simulink model "Vehicle_Performance_Model_range"  (R2020a)
settings: Solver=FixedStepAuto  StartTime=0  StopTime=50000000  FixedStep=time_step  RelTol=1e-3
values from neighbouring files (symbols this model uses):
  battery_capacity = 40000    [aa_main_code.m]
  BrkGain = 1e4    (= 10000)    [HW5_Initialization.m]    (also in aa_main_code.m; aa_main_code_optimization.m)
  Cd = 0.27    [aa_main_code.m]    (also in aa_main_code_optimization.m)
  CG_a = (mass_x_dis/mass_CG) - L104    [aa_main_code.m]    (also in aa_main_code_optimization.m)
  CG_b = L101 - CG_a    [aa_main_code.m]    (also in aa_main_code_optimization.m)
  CG_h = mass_Y_dis/mass_CG    [aa_main_code.m]    (also in aa_main_code_optimization.m)
  Cr = 0.009    [aa_main_code.m]    (also in aa_main_code_optimization.m)
  drive_ratio = 2    [aa_main_code.m]
  eff_dl = 0.9    [HW5_Initialization.m]    (also in aa_main_code.m; aa_main_code_optimization.m)
  EM_Efficiency = [0.85 0.7 0.7 0.7 0.69 0.65 0.6 0.55 0.55 0.55 0.55 0.55 ... (854 elements, 14x61)]    [MotorA_Data.mat]    (also in MotorB_Data.mat = [0.1063790939 0.270163202936 0.172582128791 0.0795422183598 ; MotorC_Data.mat = [0.156591344269 0.267837551 0.221914755199 0.160062614994 0.)
  EM_Omega_Max = [0 38.3972435439 76.7944870878 115.191730632 153.588974176 191.986217719 203.505390783 230.383461263 268.780704807 307.177948351 326.376570123 345.575191895 ... (24 elements, 1x24)]    [MotorA_Data.mat]    (also in MotorB_Data.mat = [0 334.056952995 360.213537682 388.612115341 414.768700028 4; MotorC_Data.mat = [0 130.235063563 190.672775215 254.736749566 349.019579743 3)
  EM_Torque_Max = [765 765 765 765 765 765 765 765 765 765 765 722.5 ... (24 elements, 1x24)]    [MotorA_Data.mat]    (also in MotorB_Data.mat = [300 300 279.372738239 258.745476478 241.737032569 222.55729; MotorC_Data.mat = [420 420 420 420 420 400.59405651 375.297526478 350.00099644)
  front_on = 1    [aa_main_code.m]    (also in aa_main_code_optimization.m)
  g = 9.81    [HW5_Initialization.m]    (also in aa_main_code.m; aa_main_code_optimization.m)
  Ki = 1    [HW5_Initialization.m]    (also in aa_main_code.m = 0.03; aa_main_code_optimization.m = 0.03)
  Kp = 3    [HW5_Initialization.m]    (also in aa_main_code.m = 0.5; aa_main_code_optimization.m = 0.5)
  L101 = 2700/1000    (= 2.7)    [aa_main_code.m]    (also in aa_main_code_optimization.m)
  m = 2000    [HW5_Initialization.m]
  mass = (4*passenger_mass)+cargo_mass+info_mass+sunroof_mass+unsprung_mass+total_gearbox_mass+total_differential_mass+axle_mass+body_mass+frame_rail_mass+battery_mass+total_motorinverter_mass    (= 1622.8836992)    [aa_main_code.m]    (also in aa_main_code_optimization.m = (4*passenger_mass)+cargo_mass+info_mass+sunroof_mass+unsprun)
  mu = 0.9    [HW5_Initialization.m]    (also in aa_main_code.m; aa_main_code_optimization.m)
  num_motor = 4    [aa_main_code.m]    (also in aa_main_code_optimization.m)
  omega_BP = max(size(EM_Omega_Map))    [aa_main_code.m]    (also in aa_main_code_optimization.m)
  omega_max = max(EM_Omega_Max)    [aa_main_code.m]    (also in aa_main_code_optimization.m)
  r = 0.335    [HW5_Initialization.m]    (also in aa_main_code.m = 0.32985; aa_main_code_optimization.m = 0.32985)
  rear_on = 1    [aa_main_code.m]    (also in aa_main_code_optimization.m)
  rho = 1.3    [HW5_Initialization.m]    (also in aa_main_code.m = 1.26; aa_main_code_optimization.m = 1.26)
  slope = 0.12    [aa_main_code.m]    (also in aa_main_code_optimization.m)
  torque_BP = max(size(EM_Torque_Map))    [aa_main_code.m]    (also in aa_main_code_optimization.m)
  torque_multi_factor = 2    [aa_main_code.m]    (also in aa_main_code_optimization.m)
  useful_battery_capacity = 0.95    [aa_main_code.m]    (also in aa_main_code_optimization.m)
  vehicle_frontal_area = H101*W103    (= 2.5844)    [aa_main_code.m]    (also in aa_main_code_optimization.m)
libraries: simulink x5, autolibshared x1
settings Model: Creator=palak  LastModifiedBy=atefe
settings SolverCC: AlgebraicLoopSolver=LineSearch

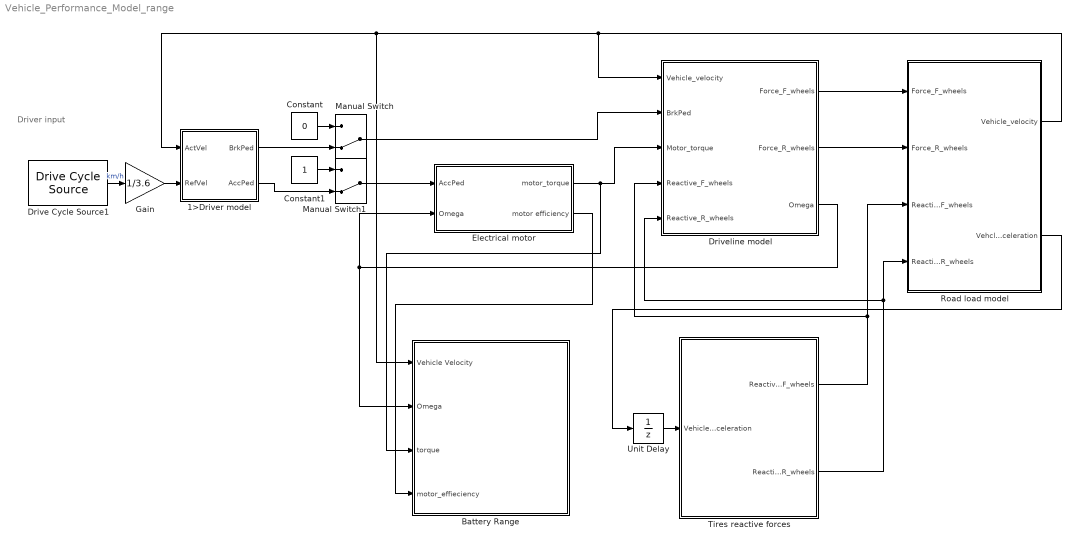
== system Vehicle_Performance_Model_range ==
  note: Driver input
  1>Driver model : Subsystem
  Battery Range : Subsystem
  Constant : Constant  Value=0
  Constant1 : Constant
  Drive Cycle Source1 : autolibshared/Drive Cycle Source  cycleVar=Workspace variable  wsVar=cycle  fileVar=cycleFTP75.mat  tfinal="600  seconds, Cyclic"  cycleRepeat=on  outAccPort=off  outGearPort=off  gearList=No gear data  t_wot1=5  xdot_woto=0  xdot_wot1=30  t_wot2=20  xdot_wot2=0  t_wotend=30  srcUnit=m/s  outUnit=m/s  srcAccUnit=m/s/s  outAccUnit=m/s^2  dt=0  aMode=1  faultOption=off  velBnd=2  velBndUnit=mph  inUnit=m/s  timeBnd=1  failOption=off  stopSim=off  maxFaultCnt=10  maxFaultTime=2  maxTotFaultTime=15  traceOption=off  dtTrace=1  traceWindow=10  lastDCname=Custom Data Set  lastOutUnit=mph  lastDT=0  lastTB=1  lastSB=2  forceCalcBound=off
      settings: SourceProductBaseCode=PW,MT,VE,VP
  Driveline model : Subsystem
  Electrical motor : Subsystem
  Gain : Gain  Gain=1/3.6
  Manual Switch : ManualSwitch  CurrentSetting=0
  Manual Switch1 : ManualSwitch  CurrentSetting=0
  Road load model : Subsystem
  Tires reactive forces : Subsystem  TreatAsAtomicUnit=on
  Unit Delay : UnitDelay  SampleTime=-1  HasFrameUpgradeWarning=on
  wires:
  Gain/1 -> 1>Driver model/2(RefVel)
  Driveline model/3(Omega) -> Electrical motor/2(Omega), Battery Range/2(Omega)
  Road load model/1(Vehicle_velocity) -> Driveline model/1(Vehicle_velocity), Battery Range/1(Vehicle Velocity), 1>Driver model/1(ActVel)
  Driveline model/1(Force_F_wheels) -> Road load model/1(Force_F_wheels)
  Manual Switch/1 -> Driveline model/2(BrkPed)
  Electrical motor/1(motor_torque) -> Battery Range/3(torque), Driveline model/3(Motor_torque)
  Road load model/2(Vehcle_acceleration) -> Unit Delay/1
  Tires reactive forces/1(Reactive_F_wheels) -> Road load model/3(Reactive_F_wheels), Driveline model/4(Reactive_F_wheels)
  Tires reactive forces/2(Reactive_R_wheels) -> Road load model/4(Reactive_R_wheels), Driveline model/5(Reactive_R_wheels)
  Driveline model/2(Force_R_wheels) -> Road load model/2(Force_R_wheels)
  Electrical motor/2(motor efficiency) -> Battery Range/4(motor_effieciency)
  Drive Cycle Source1/1 -> Gain/1  "km/h"
  Manual Switch1/1 -> Electrical motor/1(AccPed)
  1>Driver model/1(BrkPed) -> Manual Switch/2
  Constant/1 -> Manual Switch/1
  Constant1/1 -> Manual Switch1/1
  1>Driver model/2(AccPed) -> Manual Switch1/2
  Unit Delay/1 -> Tires reactive forces/1(Vehicle_acceleration)

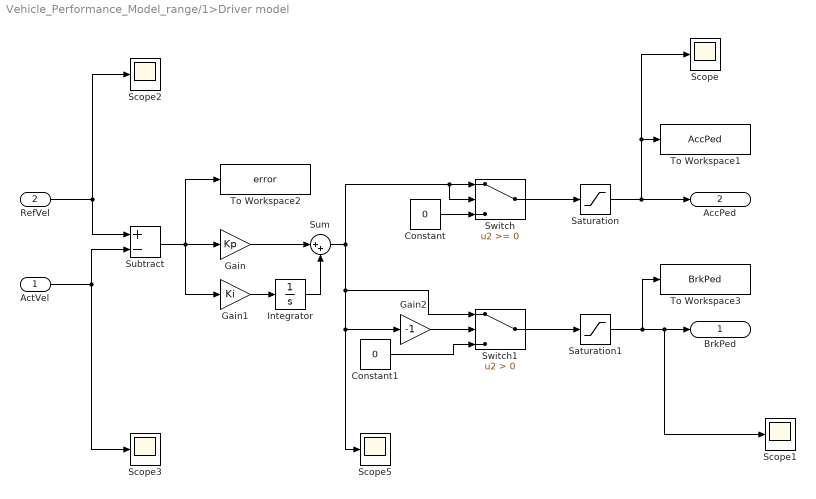
== system Vehicle_Performance_Model_range/1>Driver model ==
  ActVel : Inport  Unit=m/s
  RefVel : Inport  Port=2  Unit=m/s
  Constant : Constant  Value=0
  Constant1 : Constant  Value=0
  Gain : Gain  Gain=Kp
  Gain1 : Gain  Gain=Ki
  Gain2 : Gain  Gain=-1
  Integrator : Integrator
  Saturation : Saturate  UpperLimit=1  LowerLimit=0
  Saturation1 : Saturate  UpperLimit=0  LowerLimit=-1
  Scope{,1..3,5} (5 alike) : Scope
  Subtract : Sum  Inputs=+-
  Sum : Sum  Inputs=|++
  Switch : Switch
  Switch1 : Switch  Criteria=u2 > Threshold
  To Workspace1 : ToWorkspace  VariableName=AccPed  SaveFormat=Timeseries  SampleTime=-1
  To Workspace2 : ToWorkspace  VariableName=error  SaveFormat=Timeseries  SampleTime=-1
  To Workspace3 : ToWorkspace  VariableName=BrkPed  SaveFormat=Timeseries  SampleTime=-1
  BrkPed : Outport
  AccPed : Outport  Port=2
  wires:
  ActVel/1 -> Scope3/1, Subtract/2
  RefVel/1 -> Scope2/1, Subtract/1
  Saturation/1 -> Scope/1, To Workspace1/1, AccPed/1
  Sum/1 -> Scope5/1, Gain2/1, Switch1/1, Switch/2, Switch/1
  Subtract/1 -> Gain1/1, Gain/1, To Workspace2/1
  Gain/1 -> Sum/1
  Integrator/1 -> Sum/2
  Gain1/1 -> Integrator/1
  Constant/1 -> Switch/3
  Saturation1/1 -> Scope1/1, BrkPed/1, To Workspace3/1
  Gain2/1 -> Switch1/2
  Constant1/1 -> Switch1/3
  Switch/1 -> Saturation/1
  Switch1/1 -> Saturation1/1

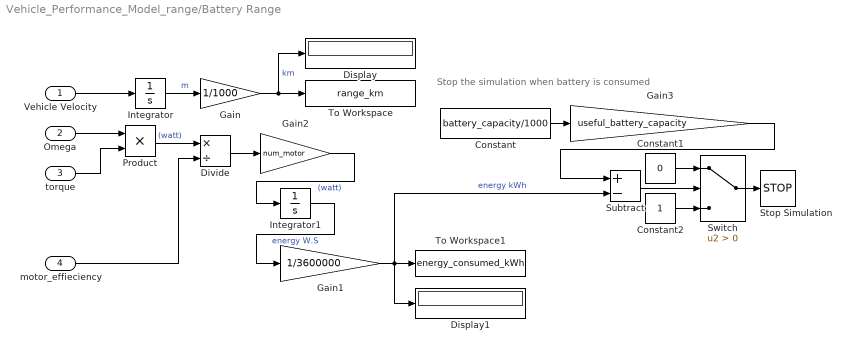
== system Vehicle_Performance_Model_range/Battery Range ==
  note: Stop the simulation when battery is consumed
  Vehicle Velocity : Inport
  Omega : Inport  Port=2
  torque : Inport  Port=3
  motor_effieciency : Inport  Port=4
  Constant : Constant  Value=battery_capacity/1000
  Constant1 : Constant  Value=0
  Constant2 : Constant
  Display : Display
  Display1 : Display
  Divide : Product  Inputs=*/
  Gain : Gain  Gain=1/1000
  Gain1 : Gain  Gain=1/3600000
  Gain2 : Gain  Gain=num_motor
  Gain3 : Gain  Gain=useful_battery_capacity
  Integrator : Integrator
  Integrator1 : Integrator
  Product : Product
  Stop Simulation : Stop
  Subtract : Sum  Inputs=+-
  Switch : Switch  Criteria=u2 > Threshold
  To Workspace : ToWorkspace  VariableName=range_km  SaveFormat=Timeseries  SampleTime=-1
  To Workspace1 : ToWorkspace  VariableName=energy_consumed_kWh  SaveFormat=Timeseries  SampleTime=-1
  wires:
  Vehicle Velocity/1 -> Integrator/1
  Gain/1 -> To Workspace/1, Display/1  "km"
  Omega/1 -> Product/1
  torque/1 -> Product/2
  Gain2/1 -> Integrator1/1  "(watt)"
  Gain1/1 -> To Workspace1/1, Subtract/2, Display1/1  "energy kWh"
  Integrator/1 -> Gain/1  "m"
  Integrator1/1 -> Gain1/1  "energy W.S"
  Product/1 -> Divide/1  "(watt)"
  Constant/1 -> Gain3/1
  Subtract/1 -> Switch/2
  Constant1/1 -> Switch/1
  Constant2/1 -> Switch/3
  Switch/1 -> Stop Simulation/1
  Gain3/1 -> Subtract/1
  motor_effieciency/1 -> Divide/2
  Divide/1 -> Gain2/1

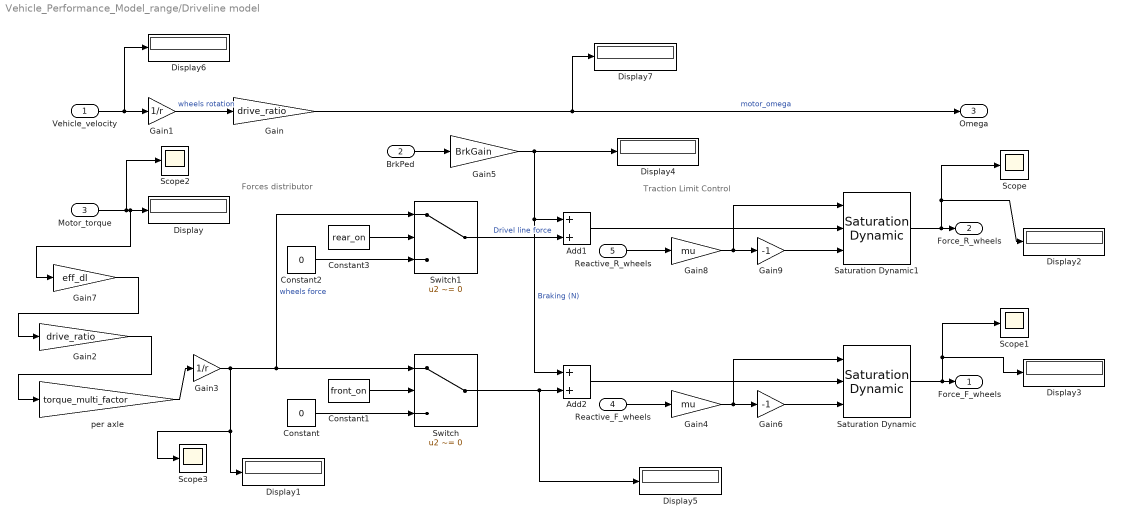
== system Vehicle_Performance_Model_range/Driveline model ==
  note: Traction Limit Control
  note: Forces distributor
  Vehicle_velocity : Inport  Unit=m/s
  BrkPed : Inport  Port=2
  Motor_torque : Inport  Port=3  Unit=N*m
  Reactive_F_wheels : Inport  Port=4  Unit=N
  Reactive_R_wheels : Inport  Port=5  Unit=N
  Add1 : Sum
  Add2 : Sum
  Constant : Constant  Value=0
  Constant1 : Constant  Value=front_on
  Constant2 : Constant  Value=0
  Constant3 : Constant  Value=rear_on
  Display{,1..7} (8 alike) : Display
  Gain : Gain  Gain=drive_ratio
  Gain1 : Gain  Gain=1/r
  Gain2 : Gain  Gain=drive_ratio
  Gain3 : Gain  Gain=1/r
  Gain4 : Gain  Gain=mu
  Gain5 : Gain  Gain=BrkGain
  Gain6 : Gain  Gain=-1
  Gain7 : Gain  Gain=eff_dl
  Gain8 : Gain  Gain=mu
  Gain9 : Gain  Gain=-1
  Saturation Dynamic : simulink/Discontinuities/Saturation Dynamic  OutMin=[]  OutMax=[]  OutDataTypeStr=Inherit: Same as second input  OutDataType=fixdt(1, 16)  OutScaling=2^-10  DoSatur=off
  Saturation Dynamic1 : simulink/Discontinuities/Saturation Dynamic  OutMin=[]  OutMax=[]  OutDataTypeStr=Inherit: Same as second input  OutDataType=fixdt(1, 16)  OutScaling=2^-10  DoSatur=off
  Scope{,1..3} (4 alike) : Scope
  Switch : Switch  Criteria=u2 ~= 0
  Switch1 : Switch  Criteria=u2 ~= 0
  per axle : Gain  Gain=torque_multi_factor
  Force_F_wheels : Outport  Unit=N
  Force_R_wheels : Outport  Port=2  Unit=N
  Omega : Outport  Port=3  Unit=rad/s
  wires:
  Gain1/1 -> Gain/1  "wheels rotation"
  Vehicle_velocity/1 -> Display6/1, Gain1/1
  Gain7/1 -> Gain2/1
  Gain2/1 -> per axle/1
  Gain3/1 -> Scope3/1, Display1/1, Switch1/1, Switch/1  "wheels force"
  BrkPed/1 -> Gain5/1
  Motor_torque/1 -> Scope2/1, Gain7/1, Display/1
  Gain5/1 -> Add2/1, Add1/1, Display4/1  "Braking (N)"
  Saturation Dynamic/1 -> Display3/1, Scope1/1, Force_F_wheels/1
  Reactive_F_wheels/1 -> Gain4/1
  Gain4/1 -> Saturation Dynamic/1, Gain6/1
  Gain6/1 -> Saturation Dynamic/3
  Add1/1 -> Saturation Dynamic1/2
  Gain8/1 -> Saturation Dynamic1/1, Gain9/1
  Gain9/1 -> Saturation Dynamic1/3
  Saturation Dynamic1/1 -> Scope/1, Display2/1, Force_R_wheels/1
  Reactive_R_wheels/1 -> Gain8/1
  Constant/1 -> Switch/3
  Constant1/1 -> Switch/2
  Add2/1 -> Saturation Dynamic/2
  Constant3/1 -> Switch1/2
  Constant2/1 -> Switch1/3
  Switch1/1 -> Add1/2  "Drivel line force"
  Switch/1 -> Display5/1, Add2/2
  Gain/1 -> Display7/1, Omega/1  "motor_omega"
  per axle/1 -> Gain3/1

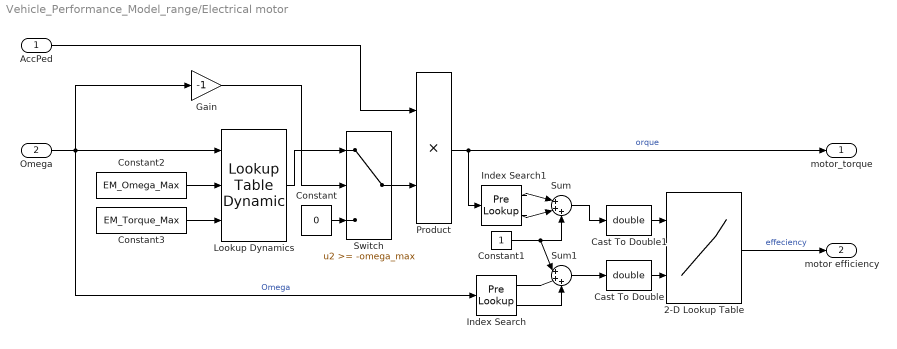
== system Vehicle_Performance_Model_range/Electrical motor ==
  AccPed : Inport
  Omega : Inport  Port=2
  2-D Lookup Table : Lookup_n-D  BreakpointsSpecification=Even spacing  BreakpointsForDimension1=[1:torque_BP]  BreakpointsForDimension2=[1:omega_BP]  Table=EM_Efficiency  ExtrapMethod=Clip  UseLastTableValue=on  InternalRulePriority=Speed  RndMeth=Simplest  InputSameDT=on
  Cast To Double : DataTypeConversion  OutDataTypeStr=double
  Cast To Double1 : DataTypeConversion  OutDataTypeStr=double
  Constant : Constant  Value=0
  Constant1 : Constant
  Constant2 : Constant  Value=EM_Omega_Max
  Constant3 : Constant  Value=EM_Torque_Max
  Gain : Gain  Gain=-1
  Index Search : PreLookup  BreakpointsData=EM_Omega_Map  IndexSearchMethod=Linear search  BreakpointDataTypeStr=double  IndexDataTypeStr=int8  RndMeth=Nearest
  Index Search1 : PreLookup  BreakpointsData=EM_Torque_Map  IndexSearchMethod=Linear search  BreakpointDataTypeStr=double  IndexDataTypeStr=int8
  Lookup Dynamics : simulink/Lookup Tables/Lookup Table Dynamic  LookUpMeth=Interpolation-Use End Values  OutDataType=fixdt('double')  OutScaling=[]  OutputDataTypeScalingMode=Specify via dialog  OutDataTypeStr=double  DoSatur=on
  Product : Product
  Sum : Sum  Inputs=|+++
  Sum1 : Sum  Inputs=|+++
  Switch : Switch  Threshold=-omega_max
  motor_torque : Outport  Unit=N*m
  motor efficiency : Outport  Port=2  Unit=N*m
  wires:
  Constant2/1 -> Lookup Dynamics/2
  Constant3/1 -> Lookup Dynamics/3
  AccPed/1 -> Product/1
  Index Search/1 -> Sum1/2
  Product/1 -> motor_torque/1, Index Search1/1  "orque"
  Cast To Double/1 -> 2-D Lookup Table/2
  Omega/1 -> Gain/1, Lookup Dynamics/1, Index Search/1  "Omega"
  Cast To Double1/1 -> 2-D Lookup Table/1
  Sum/1 -> Cast To Double1/1
  2-D Lookup Table/1 -> motor efficiency/1  "effeciency"
  Constant/1 -> Switch/3
  Switch/1 -> Product/2
  Gain/1 -> Switch/2
  Lookup Dynamics/1 -> Switch/1
  Index Search1/1 -> Sum/1
  Index Search1/2 -> Sum/2
  Constant1/1 -> Sum/3, Sum1/1
  Index Search/2 -> Sum1/3
  Sum1/1 -> Cast To Double/1

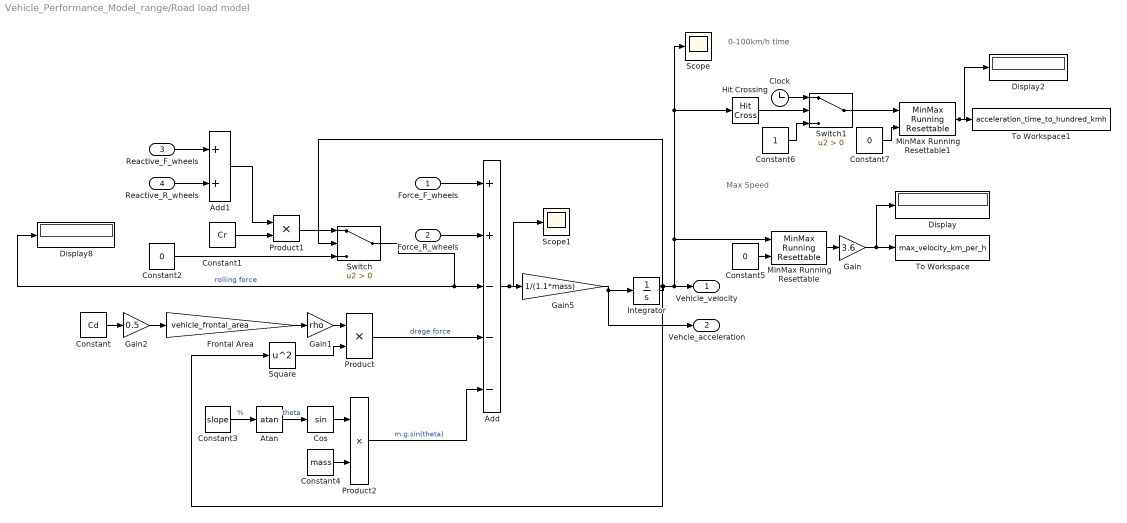
== system Vehicle_Performance_Model_range/Road load model ==
  note: 0-100km/h time
  note: Max Speed
  Force_F_wheels : Inport  Unit=N
  Force_R_wheels : Inport  Port=2  Unit=N
  Reactive_F_wheels : Inport  Port=3  Unit=N
  Reactive_R_wheels : Inport  Port=4  Unit=N
  Add : Sum  Inputs=++---
  Add1 : Sum
  Atan : Trigonometry  Operator=atan
  Clock : Clock
  Constant : Constant  Value=Cd
  Constant1 : Constant  Value=Cr
  Constant2 : Constant  Value=0
  Constant3 : Constant  Value=slope
  Constant4 : Constant  Value=mass
  Constant5 : Constant  Value=0
  Constant6 : Constant
  Constant7 : Constant  Value=0
  Cos : Trigonometry
  Display : Display
  Display2 : Display
  Display8 : Display
  Frontal Area : Gain  Gain=vehicle_frontal_area
  Gain : Gain  Gain=3.6
  Gain1 : Gain  Gain=rho
  Gain2 : Gain  Gain=0.5
  Gain5 : Gain  Gain=1/(1.1*mass)
  Hit Crossing : HitCross  HitCrossingOffset=100/3.6  HitCrossingDirection=rising
  Integrator : Integrator  LimitOutput=on  LowerSaturationLimit=0
  MinMax Running Resettable : simulink/Math Operations/MinMax Running Resettable  Function=max  vinit=0
  MinMax Running Resettable1 : simulink/Math Operations/MinMax Running Resettable  Function=max  vinit=0
  Product : Product
  Product1 : Product
  Product2 : Product
  Scope : Scope
  Scope1 : Scope
  Square : Math  Operator=square  SaturateOnIntegerOverflow=on
  Switch : Switch  Criteria=u2 > Threshold
  Switch1 : Switch  Criteria=u2 > Threshold
  To Workspace : ToWorkspace  VariableName=max_velocity_km_per_h  SaveFormat=Timeseries  SampleTime=-1
  To Workspace1 : ToWorkspace  VariableName=acceleration_time_to_hundred_kmh  SaveFormat=Timeseries  SampleTime=-1
  Vehicle_velocity : Outport  Unit=m/s
  Vehcle_acceleration : Outport  Port=2  Unit=m/s
  wires:
  Constant/1 -> Gain2/1
  Frontal Area/1 -> Gain1/1
  Gain2/1 -> Frontal Area/1
  Gain1/1 -> Product/1
  Product/1 -> Add/4  "drage force"
  Switch/1 -> Display8/1, Add/3  "rolling force"
  Force_F_wheels/1 -> Add/1
  Add/1 -> Scope1/1, Gain5/1
  Gain5/1 -> Integrator/1, Vehcle_acceleration/1
  Square/1 -> Product/2
  Constant2/1 -> Switch/3
  Constant1/1 -> Product1/2
  Force_R_wheels/1 -> Add/2
  Reactive_F_wheels/1 -> Add1/1
  Reactive_R_wheels/1 -> Add1/2
  Add1/1 -> Product1/1
  Product1/1 -> Switch/1
  Cos/1 -> Product2/1
  Atan/1 -> Cos/1  "theta"
  Constant3/1 -> Atan/1  "%"
  Constant4/1 -> Product2/2
  Product2/1 -> Add/5  "m.g.sin(theta)"
  MinMax Running Resettable/1 -> Gain/1
  Constant5/1 -> MinMax Running Resettable/2
  Integrator/1 -> Switch/2, Square/1, MinMax Running Resettable/1, Scope/1, Hit Crossing/1, Vehicle_velocity/1
  Constant6/1 -> Switch1/3
  MinMax Running Resettable1/1 -> Display2/1, To Workspace1/1
  Constant7/1 -> MinMax Running Resettable1/2
  Switch1/1 -> MinMax Running Resettable1/1
  Clock/1 -> Switch1/1
  Hit Crossing/1 -> Switch1/2
  Gain/1 -> To Workspace/1, Display/1

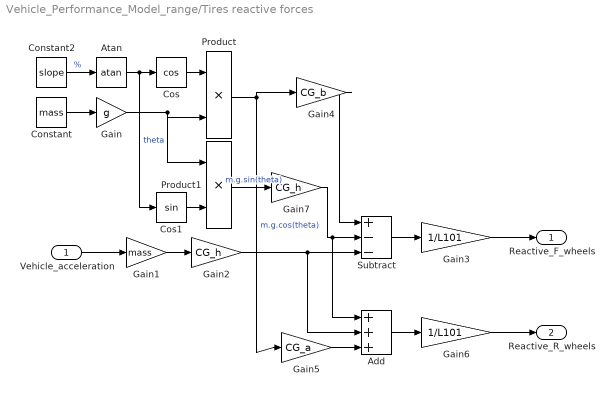
== system Vehicle_Performance_Model_range/Tires reactive forces ==
  Vehicle_acceleration : Inport
  Add : Sum  Inputs=+++
  Atan : Trigonometry  Operator=atan
  Constant : Constant  Value=mass
  Constant2 : Constant  Value=slope
  Cos : Trigonometry  Operator=cos
  Cos1 : Trigonometry
  Gain : Gain  Gain=g
  Gain1 : Gain  Gain=mass
  Gain2 : Gain  Gain=CG_h
  Gain3 : Gain  Gain=1/L101
  Gain4 : Gain  Gain=CG_b
  Gain5 : Gain  Gain=CG_a
  Gain6 : Gain  Gain=1/L101
  Gain7 : Gain  Gain=CG_h
  Product : Product
  Product1 : Product
  Subtract : Sum  Inputs=+--
  Reactive_F_wheels : Outport
  Reactive_R_wheels : Outport  Port=2
  wires:
  Constant2/1 -> Atan/1  "%"
  Atan/1 -> Cos1/1, Cos/1  "theta"
  Constant/1 -> Gain/1
  Gain/1 -> Product1/1, Product/2
  Cos/1 -> Product/1
  Vehicle_acceleration/1 -> Gain1/1
  Gain1/1 -> Gain2/1
  Gain2/1 -> Subtract/3, Add/2
  Gain4/1 -> Subtract/1
  Subtract/1 -> Gain3/1
  Gain3/1 -> Reactive_F_wheels/1
  Product/1 -> Gain5/1, Gain4/1  "m.g.cos(theta)"
  Gain5/1 -> Add/3
  Add/1 -> Gain6/1
  Gain6/1 -> Reactive_R_wheels/1
  Cos1/1 -> Product1/2
  Product1/1 -> Gain7/1  "m.g.sin(theta)"
  Gain7/1 -> Add/1, Subtract/2
